simulink library "BUS_Subsystem"  (R2016b)
settings: Solver=VariableStepAuto  StartTime=0.0  StopTime=10.0  RelTol=1e-3
libraries: BUS_IN x1, BUS_OUT x1
settings Model: Creator=Alexander Koch  LastModifiedBy=Alexander Koch

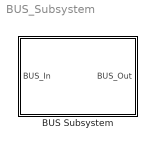
== system BUS_Subsystem ==
  BUS Subsystem : Subsystem
      mask help:
      | <Author> Alexander Koch based on Stefan Müller, Stephan Rohr
      | <Date> 03/04/2017
      |
      | <Description>
      | Consist of a Bus In and a Bus Out Block. To Select Signals from the Bus open the Bus In Block, to write signals to the Bus under a certain tab name open the bus out block. For further information, please read the discription of the Bus In and Bus out Block
      |
      | The Block automaticlly disconnects the link to the library block after opening the first time
      |
      | <Parameters>
      | -
      |
      | <Inputs>
      | BUS_In [Bus]
      |
      | <Outputs>
      | Bus_Out [Bus]
      settings: OpenFcn=|
      | set_param(gcb(),'LinkStatus','none')
      | open_system(gcb(),'force')

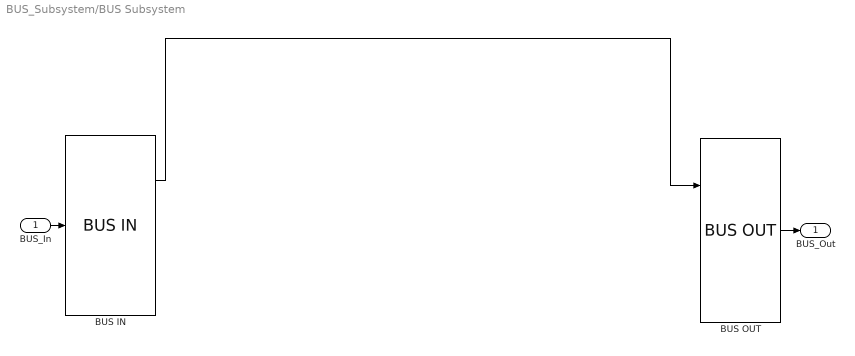
== system BUS_Subsystem/BUS Subsystem ==
  BUS_In : Inport
  BUS IN : BUS_IN/BUS IN
  BUS OUT : BUS_OUT/BUS OUT  NumberofInputs=1  NameSys='Subsystem'
  BUS_Out : Outport
  wires:
  BUS_In/1 -> BUS IN/1
  BUS OUT/1 -> BUS_Out/1
  BUS IN/1 -> BUS OUT/1
